simulink model "ARDroneFly_035"  (R2014b)
settings: Solver=FixedStepDiscrete  StartTime=0.0  StopTime=600  FixedStep=1/400  RelTol=1e-3
InitFcn:
  | AR_DRONE_SCRIPT;
  | ControllerDesign;
  | parameters;
values from neighbouring files (symbols this model uses):
  Ah = [0 1; 0 0]    [ControllerDesign.m]
  Axy = [0 1; 0 0]    [ControllerDesign.m]
  C = (eval(C))    [ControllerDesign.m]
  Ch = [1 0]    [ControllerDesign.m]
  Cxy = [1 0]    [ControllerDesign.m]
  Lh = Lh'    [ControllerDesign.m]
  Lxy = Lxy'    [ControllerDesign.m]
  par_g = par.g    [parameters.m]
  par_m = par.m    [parameters.m]
  tauToPwmbar = inv(pwmbarToTau)    [ControllerDesign.m]
undefined symbols (not defined in the file or in its folder): meter, par
libraries: simulink x6, AR_Drone_2_Library x5, dspnetwork x1
(part 1 of 2)
settings Model: SimulationMode=external  ExtModeTrigDuration=120003  Creator=darenlee  LastModifiedBy=s136047
settings OptimizationCC: OptimizeModelRefInitCode=on  LifeSpan=1  MaxStackSize=64
settings DebuggingCC: UnderspecifiedInitializationDetection=Classic  MergeDetectMultiDrivingBlocksExec=none
settings HardwareCC: ProdLargestAtomicInteger=Long  ProdLargestAtomicFloat=Double  ProdEndianess=LittleEndian  ProdHWDeviceType=ARM Compatible->ARM Cortex
settings RTWCC: SystemTargetFile=ert.tlc  TLCOptions=-aInlineSetEventsForThisBaseRateFcn=TLC_FALSE -aSuppressMultiTaskScheduler=TLC_FALSE  TemplateMakefile=ert_default_tmf  Description=Embedded Coder  ProcessScript=ert_make_rtw_hook  Toolchain=Code Sourcery
settings CodeAppCC: IgnoreCustomStorageClasses=off
settings ERTTargetCC: ExtMode=on  ExtModeMexArgs='192.168.1.1' 1 17725

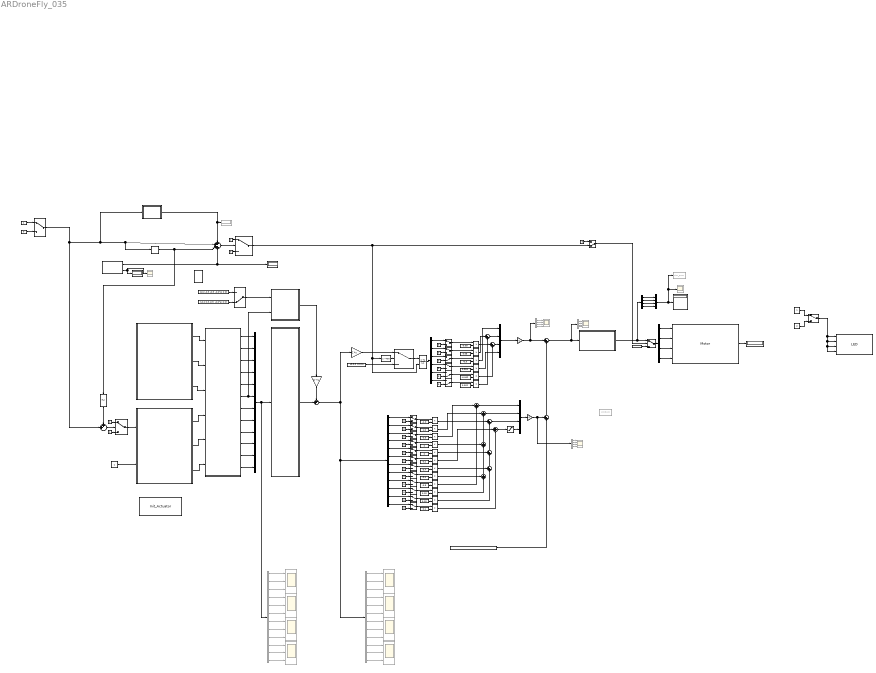
== system ARDroneFly_035 ==
  note: This version is not yet optimal, but some parts work, sorry.
      |
      | Based on: https://github.com/darenlee/SimulinkARDroneTarget
      |
      | Take off
      | 1) Make sure external camera feedback is activated in another Matlab Window (UDP Connection)
      | 2) Activate Green Manual Switch (will only take effect on rising edge)
      | 3) "Take off" signal is 2 seconds delayed, in this time the sensors are calibrated
      | 4) Quad fly's to the the setpoint (blue button)
      |
      | Stop
      | 1) Deactivate Green Manual Switch
      | 2) Quad falls out of the air
      |
      | Low voltage
      | 1) once the voltage has dropped once under the 9 volt the quad will not takeoff again
      | 2) or reset manually in the 'battery check' block
      |
      | Tips to tune the quad
      | 1) deactivate all feedback (manual switches) except for the z, roll, pitch and omega_xyz control
      | 2) test if the quad is some kind of stable (if not then change the gains) (first roll and pitch then omega_xy (omega functions as a differential action (damping)))
      | 3) try to manage that the quad takes off vertically by changing the gravity compensation term
      | 4) tune the rest of the proportional part
      | 5) activate and tune the integral part (be gentle with this one)
      | 6) have a look at the lowpass, luenberger observers (X-Y pos), and the complementary sensor fusion (accel gyro)
  note: [ T_0 TauX_0 TauY_0 TauZ_0 ]
  note: Integral action
  note: Setpoint [ x y z yaw u v ] (in inertia frame)
      | Note: Z must be negative because
      | of NED coordinates
  note: Delay is  added to
      | start integration action only
      | when quad is in the air
  note: Proportional action
  note: Gravity compensation
  0 when battery dropped once under 9 volt 1 when battery OK : Display
  Accel_Norm1 : Scope  Commented=on
      settings: ShowLegends=on  YMin=0  YMax=90  SaveName=Accel_P1
  Accel_Norm10 : Scope  Commented=on  NumInputPorts=4
      settings: ShowLegends=on  YMin=0~-1~-1~-1  YMax=20~1~1~1  SaveName=Accel_P15
  Accel_Norm{2..4,6,8..9,11..12} (8 alike) : Scope  Commented=on  NumInputPorts=3
      Accel_Norm11 settings: YMin=-0.4~-0.4~-0.5  YMax=0.2~0.4~0.2  SaveName=Accel_P2
      Accel_Norm12 settings: YMin=-0.8~-0.6~-0.4  YMax=1.2~0.6~0.4  SaveName=Accel_P7
      Accel_Norm2 settings: YMin=-0.5~-0.4~-0.235  YMax=0.3~0.5~-0.195  SaveName=Accel_P8
      Accel_Norm3 settings: YMin=-0.5~-0.4~0.25  YMax=0.5~0.5~0.5  SaveName=Accel_P
      Accel_Norm4 settings: YMin=-1~-1~-1.5  YMax=1~1~2  SaveName=Accel_P10
      Accel_Norm6 settings: YMin=-1~-1~-1.5  YMax=1~1~2  SaveName=Accel_P3
      Accel_Norm8 settings: YMin=-0.4~-0.4~-0.5  YMax=0.2~0.4~0.2  SaveName=Accel_P4
      Accel_Norm9 settings: YMin=-0.8~-0.6~-0.4  YMax=1.2~0.6~0.4  SaveName=Accel_P6
  Accel_Norm13 : Scope  Commented=on  NumInputPorts=4
      settings: ShowLegends=on  YMin=-0.5~-0.15~-0.15~-0.2  YMax=0.2~0.1~0.15~0.2  SaveName=Accel_P18
  Accel_Norm14 : Scope  Commented=on  NumInputPorts=4
      settings: ShowLegends=on  YMin=3.7~-0.25~-0.5~-0.15  YMax=4.2~0.1~1.5~0.05  SaveName=Accel_P19
  Accel_Norm7 : Scope  Commented=on
      settings: YMin=9  YMax=12  SaveName=Accel_P11
  Battery Check : Subsystem
  Constant{,7..8,10,57} (5 alike) : Constant
  Constant1 : Constant  Value=2
  Constant{5,9,12,30,39..53,56,59,61} (22 alike) : Constant  Value=0
  Constant13 : Constant  Value=[0 0 0 0]
  Constant14 : Constant  Value=-1.0
  Constant15 : Constant  Value=1.0
  Constant16 : Constant  Value=-0.9
  Constant17 : Constant  Value="[-0.2 -0.3 -0.5  -0.0*pi 0 0]"
  Constant2 : Constant  Value=0.4
  Constant20 : Constant  Value=2
  Constant21 : Constant  Value=2
  Constant22 : Constant  Value=0.2
  Constant23 : Constant  Value=-0.4
  Constant24 : Constant  Value="[1.1*par_m*par_g      -0.02     -0.083    -0.027]"
  Constant27 : Constant  Value=-0.05
  Constant28 : Constant  Value=0.05
  Constant29 : Constant  Value=-0.5
  Constant3 : Constant  Value="[-0.2 0.3 -0.5  -0.0*pi 0 0]"
  Constant32 : Constant  Value=0.004
  Constant33 : Constant  Value=0.15
  Constant34 : Constant  Value=0.15
  Constant35 : Constant  Value=0.1
  Constant58 : Constant  Value=-0.002
  Constant6 : Constant  Value=-0.5
  Constant60 : Constant  Value=0.002
  Constant62 : Constant  Value="[0 0 0  0 0 0]"
  Delay1 : Delay  DelayLength=800  InitialCondition=0
  Delay3 : Delay  DelayLength=400  InitialCondition=0
  Demux1 : Demux  Commented=on  Outputs=12
  Demux10 : Demux  Commented=on
  Demux11 : Demux  Commented=on
  Demux12 : Demux  Commented=on
  Demux3 : Demux  Commented=on  Outputs=12
  Demux4 : Demux
  Demux5 : Demux
  Demux8 : Demux  Outputs=12
  Demux9 : Demux  Outputs=6
  Discrete-Time Integrator1 : DiscreteIntegrator  ExternalReset=rising  InitialConditionSetting=State (most efficient)  SampleTime=-1
  Gain2 : Gain  Gain=C'  Multiplication=Matrix(K*u)
  Gain6 : Gain  Gain=C  Multiplication=Matrix(K*u)  SampleTime=0.0025
  Init_Actuator : AR_Drone_2_Library/Init_Actuator  ShowSpec=on
  Invert Signal : Fcn  Expr=-(u(1)-1)
  LED : AR_Drone_2_Library/LED
  Low Pass Filters and Luenberg Observers : Subsystem
  Mag1 : Display
  Manual Switch{3..16,18} (15 alike) : ManualSwitch
  Manual Switch{17,19..21} (4 alike) : ManualSwitch  CurrentSetting=0
  Motor : AR_Drone_2_Library/Motor
  Motor Thrust/Torque model : Subsystem
  Mux14 : Mux
  Mux15 : Mux
  Mux4 : Mux  Inputs=12
  Mux6 : Mux
  Negative gain feedback : Gain  Gain=-1
  Negative integral feedback : Gain  Gain=-1
  Product{1..3,7..10,12..22} (18 alike) : Product
  "Sensor Measurements, Low Pass Filter, Calibrations, and Corrections " : Subsystem
  Set and hold after first rising edge : Subsystem
  Setpoint To Pilot Frame : Subsystem
  "Shut off pwm output (debug purpose) " : ManualSwitch  CurrentSetting=0
  States To Pilot Frame : Subsystem
  Sum{1..2,5,10,12,16,22} (7 alike) : Sum  Inputs=|++
  Sum{8,17..21} (6 alike) : Sum  Inputs=++|
  Sum3 : Sum  Inputs=++++
  Sum7 : Sum  Inputs=-+|
  Switch : Switch  Criteria=u2 > Threshold
  Switch1 : Switch  Threshold=4
  Switch3 : Switch  Threshold=2
  Switch4 : Switch  Threshold=1
  Switch6 : Switch  Criteria=u2 > Threshold
  Take off and shutdown (reacts only at rising edges) : ManualSwitch
  To Workspace4 : ToWorkspace  Commented=on  VariableName=simPwm  SampleTime=-1
  To Workspace7 : ToWorkspace  Commented=on  VariableName=sim_pwm  SaveFormat=Timeseries  SampleTime=-1
  Volt : Display
  Volt3 : Display  Commented=on
  We lost too much thrust if we dont do this (gain too high) : Saturate  UpperLimit=0.1  LowerLimit=-0.1
  from topcam via UDP : Subsystem
  track yaw : Subsystem
  ydf1 : Display
  wires:
  Switch/1 -> LED/4, LED/3, LED/2, LED/1
  Motor/1 -> Mag1/1
  Switch3/1 -> "Sensor Measurements, Low Pass Filter, Calibrations, and Corrections "/1(Hold Calibration Signal)
  Constant7/1 -> "Sensor Measurements, Low Pass Filter, Calibrations, and Corrections "/2(Activate Calibration Accel Angles)
  Switch1/1 -> Discrete-Time Integrator1/2, Delay3/1, "Shut off pwm output (debug purpose) "/2
  Constant5/1 -> Switch1/3
  Constant8/1 -> Switch1/1
  Constant9/1 -> Take off and shutdown (reacts only at rising edges)/2
  Constant10/1 -> Take off and shutdown (reacts only at rising edges)/1
  Sum3/1 -> Switch1/2
  Battery Check/1(Battery Volt OK) -> 0 when battery dropped once under 9 volt 1 when battery OK/1, Sum3/4
  Battery Check/2(volt) -> Volt/1, Accel_Norm7/1
  Demux4/2 -> Mux6/2  "2"
  Demux4/1 -> Mux6/1  "1"
  Demux4/3 -> Mux6/3  "3"
  Demux4/4 -> Mux6/4  "4"
  Mux6/1 -> To Workspace7/1, Accel_Norm1/1, ydf1/1
  "Shut off pwm output (debug purpose) "/1 -> Switch6/2
  Constant12/1 -> "Shut off pwm output (debug purpose) "/1
  Switch6/1 -> Demux5/1
  Constant13/1 -> Switch6/3
  Demux5/4 -> Motor/4  "4"
  Demux5/3 -> Motor/3  "3"
  Demux5/2 -> Motor/2  "2"
  Demux5/1 -> Motor/1  "1"
  "Sensor Measurements, Low Pass Filter, Calibrations, and Corrections "/2(Roll Pitch (Integrated Gyro + Accel Corrected)) -> Low Pass Filters and Luenberg Observers/5(roll pitch_in)
  "Sensor Measurements, Low Pass Filter, Calibrations, and Corrections "/3(Gyro omega_xyz) -> Low Pass Filters and Luenberg Observers/6(wx wy wz_ in)
  "Sensor Measurements, Low Pass Filter, Calibrations, and Corrections "/1(Height UltraSound) -> Low Pass Filters and Luenberg Observers/4(z_in)
  Constant14/1 -> Product1/2
  Constant15/1 -> Product2/2
  Constant16/1 -> Product3/2
  Constant20/1 -> Product7/2
  Constant21/1 -> Product8/2
  Constant22/1 -> Product9/2
  Constant23/1 -> Product10/2
  Sum1/1 -> Mux14/1  "T"
  Sum5/1 -> Mux14/3  "tau_y"
  Sum2/1 -> Mux14/2  "tau_x"
  Mux14/1 -> Negative gain feedback/1
  Constant24/1 -> Sum20/2
  Constant27/1 -> Product12/2
  Constant28/1 -> Product13/2
  Constant29/1 -> Product14/2
  Discrete-Time Integrator1/1 -> Demux9/1
  Sum20/1 -> Sum12/2
  Sum12/1 -> Motor Thrust/Torque model/1("[ T tau_xyz ]"), Demux12/1
  Mux15/1 -> Negative integral feedback/1
  Constant32/1 -> Product15/2
  Negative integral feedback/1 -> Sum12/1, Demux10/1
  Demux10/1 -> Accel_Norm10/1
  Demux10/4 -> Accel_Norm10/4
  Demux10/3 -> Accel_Norm10/3
  Demux10/2 -> Accel_Norm10/2
  Negative gain feedback/1 -> Demux11/1, Sum20/1
  Demux11/1 -> Accel_Norm13/1
  Demux11/4 -> Accel_Norm13/4
  Demux11/3 -> Accel_Norm13/3
  Demux11/2 -> Accel_Norm13/2
  Demux12/1 -> Accel_Norm14/1
  Demux12/4 -> Accel_Norm14/4
  Demux12/3 -> Accel_Norm14/3
  Demux12/2 -> Accel_Norm14/2
  from topcam via UDP/1(real x) -> Low Pass Filters and Luenberg Observers/1(x_in)
  from topcam via UDP/2("real y ") -> Low Pass Filters and Luenberg Observers/2(y_in)
  from topcam via UDP/3(real psi) -> Low Pass Filters and Luenberg Observers/3(yaw_in)
  Constant2/1 -> Product17/2
  Constant6/1 -> Product18/2
  Constant33/1 -> Product19/2
  Constant34/1 -> Product20/2
  Constant35/1 -> Product16/2
  Demux8/2 -> Manual Switch4/1  "y"
  Demux8/3 -> Manual Switch5/1  "z"
  Demux8/1 -> Manual Switch3/1  "x"
  Demux8/6 -> Manual Switch8/1  "yaw"
  Sum16/1 -> We lost too much thrust if we dont do this (gain too high)/1
  Product18/1 -> Sum1/2
  Product19/1 -> Sum17/2
  Product17/1 -> Sum17/1
  Product20/1 -> Sum18/2
  Product10/1 -> Sum18/1  "tau_z"
  Product9/1 -> Sum16/1
  Product1/1 -> Sum5/1
  Product2/1 -> Sum2/1
  Product3/1 -> Sum1/1
  Sum19/1 -> Sum2/2
  Sum17/1 -> Sum19/2
  Product7/1 -> Sum19/1
  Sum21/1 -> Sum5/2
  Sum18/1 -> Sum21/2
  Product8/1 -> Sum21/1
  Manual Switch3/1 -> Product1/1
  Constant39/1 -> Manual Switch3/2
  Constant40/1 -> Manual Switch4/2
  Constant41/1 -> Manual Switch5/2
  Constant42/1 -> Manual Switch6/2
  Constant43/1 -> Manual Switch7/2
  Constant44/1 -> Manual Switch8/2
  Constant45/1 -> Manual Switch9/2
  Constant46/1 -> Manual Switch10/2
  Constant47/1 -> Manual Switch11/2
  Constant48/1 -> Manual Switch12/2
  Constant49/1 -> Manual Switch13/2
  Constant50/1 -> Manual Switch14/2
  Demux8/12 -> Manual Switch14/1  "omega z"
  Demux8/11 -> Manual Switch13/1  "omega y"
  Demux8/10 -> Manual Switch12/1  "omega x"
  Demux8/9 -> Manual Switch11/1  "w"
  Demux8/8 -> Manual Switch10/1  "v"
  Demux8/7 -> Manual Switch9/1  "u"
  Demux8/5 -> Manual Switch7/1  "pitch"
  Demux8/4 -> Manual Switch6/1  "roll"
  Manual Switch14/1 -> Product16/1
  Manual Switch13/1 -> Product20/1
  Manual Switch12/1 -> Product19/1
  Manual Switch11/1 -> Product18/1
  Manual Switch10/1 -> Product17/1
  Manual Switch9/1 -> Product10/1
  Manual Switch8/1 -> Product9/1
  Manual Switch7/1 -> Product8/1
  Manual Switch6/1 -> Product7/1
  Manual Switch5/1 -> Product3/1
  Manual Switch4/1 -> Product2/1
  Product14/1 -> Mux15/1  "T"
  Product15/1 -> Mux15/4  "tau_z"
  Constant30/1 -> Manual Switch15/2
  Constant51/1 -> Manual Switch16/2
  Constant52/1 -> Manual Switch17/2
  Constant53/1 -> Manual Switch18/2
  Manual Switch18/1 -> Product15/1
  Demux9/4 -> Manual Switch18/1  "yaw"
  Manual Switch17/1 -> Product14/1
  Demux9/3 -> Manual Switch17/1  "z"
  Demux9/2 -> Manual Switch16/1  "y"
  Manual Switch16/1 -> Product13/1
  Manual Switch15/1 -> Product12/1
  Demux9/1 -> Manual Switch15/1  "x"
  Constant1/1 -> Switch/3
  Constant/1 -> Switch/1
  Delay1/1 -> Sum3/3, Invert Signal/1
  Constant56/1 -> Switch3/1
  Constant57/1 -> Switch3/3
  Set and hold after first rising edge/1(Out) -> Volt3/1, Sum3/1
  Take off and shutdown (reacts only at rising edges)/1 -> Sum8/2, Delay1/1, Sum3/2, Set and hold after first rising edge/1(In)
  Constant58/1 -> Product21/2
  Constant59/1 -> Manual Switch19/2
  Manual Switch19/1 -> Product21/1
  Demux9/5 -> Manual Switch19/1  "u"
  Constant60/1 -> Product22/2
  Constant61/1 -> Manual Switch20/2
  Manual Switch20/1 -> Product22/1
  Demux9/6 -> Manual Switch20/1  "v"
  Sum10/1 -> Mux15/3  "tau_y"
  Product12/1 -> Sum10/1  "tau_y"
  Product21/1 -> Sum10/2
  Sum22/1 -> Mux15/2  "tau_x"
  Product13/1 -> Sum22/1  "tau_x"
  Product22/1 -> Sum22/2
  Switch4/1 -> Discrete-Time Integrator1/1
  Sum8/1 -> Switch3/2
  Invert Signal/1 -> Sum8/1
  Delay3/1 -> Switch4/2
  Demux1/1 -> Accel_Norm3/1
  Demux1/2 -> Accel_Norm3/2
  Demux1/3 -> Accel_Norm3/3
  Demux1/4 -> Accel_Norm6/1
  Demux1/5 -> Accel_Norm6/2
  Demux1/6 -> Accel_Norm6/3
  Demux1/7 -> Accel_Norm8/1
  Demux1/8 -> Accel_Norm8/2
  Demux1/9 -> Accel_Norm8/3
  Demux1/10 -> Accel_Norm9/1
  Demux1/11 -> Accel_Norm9/2
  Demux1/12 -> Accel_Norm9/3
  Low Pass Filters and Luenberg Observers/1(x_out) -> Mux4/1
  Low Pass Filters and Luenberg Observers/2(y_out) -> Mux4/2
  Low Pass Filters and Luenberg Observers/3(z_out) -> Mux4/3
  Low Pass Filters and Luenberg Observers/4(roll_out) -> Mux4/4
  Low Pass Filters and Luenberg Observers/5(pitch_out) -> Mux4/5
  Low Pass Filters and Luenberg Observers/6(yaw out) -> Setpoint To Pilot Frame/2(yaw), Mux4/6
  Low Pass Filters and Luenberg Observers/7(u_out) -> Mux4/7
  Low Pass Filters and Luenberg Observers/8(v_out) -> Mux4/8
  Low Pass Filters and Luenberg Observers/9(w_out) -> Mux4/9
  Low Pass Filters and Luenberg Observers/10(omega x_out) -> Mux4/10
  Low Pass Filters and Luenberg Observers/11(omega y_out) -> Mux4/11
  Low Pass Filters and Luenberg Observers/12(omega z_out) -> Mux4/12
  Mux4/1 -> Demux3/1, States To Pilot Frame/1(State)
  Gain6/1 -> Switch4/1
  Constant62/1 -> Switch4/3
  Demux3/1 -> Accel_Norm2/1
  Demux3/2 -> Accel_Norm2/2
  Demux3/3 -> Accel_Norm2/3
  Demux3/4 -> Accel_Norm4/1
  Demux3/5 -> Accel_Norm4/2
  Demux3/6 -> Accel_Norm4/3
  Demux3/7 -> Accel_Norm11/1
  Demux3/8 -> Accel_Norm11/2
  Demux3/9 -> Accel_Norm11/3
  Demux3/10 -> Accel_Norm12/1
  Demux3/11 -> Accel_Norm12/2
  Demux3/12 -> Accel_Norm12/3
  States To Pilot Frame/1(State pilot frame) -> Sum7/2
  Gain2/1 -> Sum7/1
  Setpoint To Pilot Frame/1(Setpoint pilot frame) -> Gain2/1
  Sum7/1 -> Demux1/1, Demux8/1, Gain6/1  "Error Signal"
  Product16/1 -> Sum16/2
  We lost too much thrust if we dont do this (gain too high)/1 -> Mux14/4
  Motor Thrust/Torque model/1(PWM_1,2,3,4) -> Switch6/1, Demux4/1
  Constant17/1 -> Manual Switch21/1
  Constant3/1 -> Manual Switch21/2
  Manual Switch21/1 -> Setpoint To Pilot Frame/1(Setpoint)

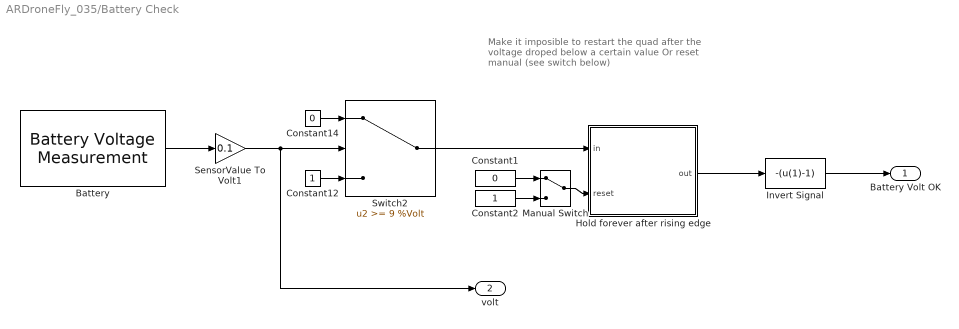
== system ARDroneFly_035/Battery Check ==
  note: Make it imposible to restart the quad
      | after the voltage droped below a certain value
      |
      | Or reset manual (see switch below)
  Battery : AR_Drone_2_Library/Battery Voltage Measurement  SFunctionSpec=void BatteryMeasure_step(single y1[1])  SampleTime=-1
  Constant1 : Constant  Value=0
  Constant12 : Constant
  Constant14 : Constant  Value=0
  Constant2 : Constant
  Hold forever after rising edge : Subsystem
  Invert Signal : Fcn  Expr=-(u(1)-1)
  Manual Switch : ManualSwitch
  SensorValue To Volt1 : Gain  Gain=0.1
  Switch2 : Switch  Threshold=9 %Volt
  Battery Volt OK : Outport
  volt : Outport  Port=2
  wires:
  Constant14/1 -> Switch2/1
  Constant12/1 -> Switch2/3
  Battery/1 -> SensorValue To Volt1/1
  SensorValue To Volt1/1 -> volt/1, Switch2/2
  Switch2/1 -> Hold forever after rising edge/1(in)
  Hold forever after rising edge/1(out) -> Invert Signal/1
  Constant1/1 -> Manual Switch/1
  Constant2/1 -> Manual Switch/2
  Manual Switch/1 -> Hold forever after rising edge/2(reset)
  Invert Signal/1 -> Battery Volt OK/1

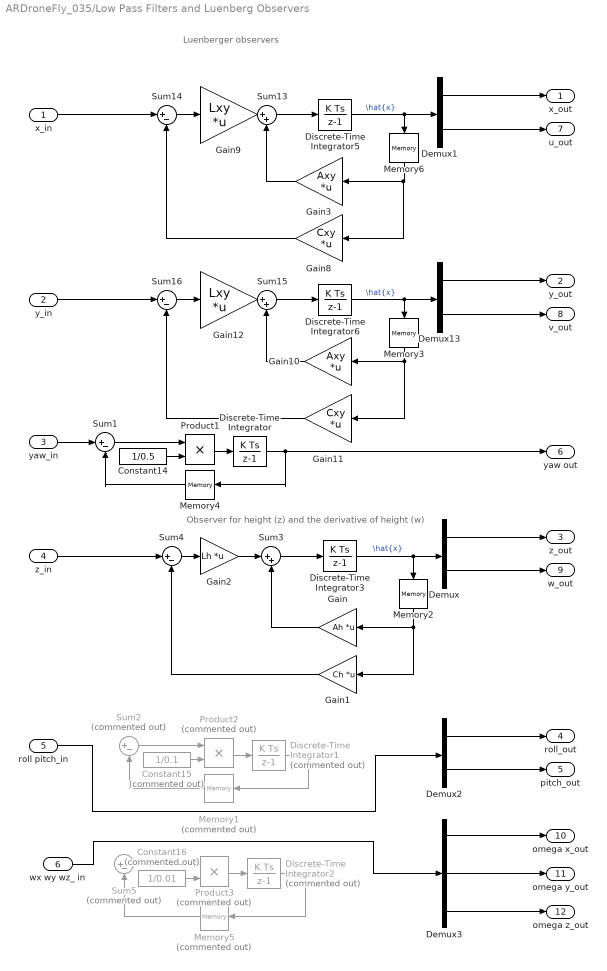
== system ARDroneFly_035/Low Pass Filters and Luenberg Observers ==
  note: Luenberger observers
  note: Observer for height (z) and the derivative of height (w)
  x_in : Inport
  y_in : Inport  Port=2
  yaw_in : Inport  Port=3
  z_in : Inport  Port=4
  roll pitch_in : Inport  Port=5
  wx wy wz_ in : Inport  Port=6
  Constant14 : Constant  Value=1/0.5
  Constant15 : Constant  Commented=on  Value=1/0.1
  Constant16 : Constant  Commented=on  Value=1/0.01
  Demux{,1..2,13} (4 alike) : Demux  Outputs=2
  Demux3 : Demux  Outputs=3
  Discrete-Time Integrator : DiscreteIntegrator  InitialConditionSetting=State (most efficient)  SampleTime=-1
  Discrete-Time Integrator1 : DiscreteIntegrator  Commented=on  InitialConditionSetting=State (most efficient)  SampleTime=-1
  Discrete-Time Integrator2 : DiscreteIntegrator  Commented=on  InitialConditionSetting=State (most efficient)  SampleTime=-1
  Discrete-Time Integrator3 : DiscreteIntegrator  InitialCondition=[0 0]  InitialConditionSetting=State (most efficient)  SampleTime=-1
  Discrete-Time Integrator5 : DiscreteIntegrator  InitialCondition=[0 0]  InitialConditionSetting=State (most efficient)  SampleTime=-1
  Discrete-Time Integrator6 : DiscreteIntegrator  InitialCondition=[0 0]  InitialConditionSetting=State (most efficient)  SampleTime=-1
  Gain : Gain  Gain=Ah  Multiplication=Matrix(K*u)
  Gain1 : Gain  Gain=Ch  Multiplication=Matrix(K*u)
  Gain10 : Gain  Gain=Axy  Multiplication=Matrix(K*u)
  Gain11 : Gain  Gain=Cxy  Multiplication=Matrix(K*u)
  Gain12 : Gain  Gain=Lxy  Multiplication=Matrix(K*u)
  Gain2 : Gain  Gain=Lh  Multiplication=Matrix(K*u)
  Gain3 : Gain  Gain=Axy  Multiplication=Matrix(K*u)
  Gain8 : Gain  Gain=Cxy  Multiplication=Matrix(K*u)
  Gain9 : Gain  Gain=Lxy  Multiplication=Matrix(K*u)
  Memory1 : Memory  Commented=on
  Memory{2..4,6} (4 alike) : Memory
  Memory5 : Memory  Commented=on
  Product1 : Product
  Product2 : Product  Commented=on
  Product3 : Product  Commented=on
  Sum{1,4,14,16} (4 alike) : Sum  Inputs=|+-
  Sum13 : Sum  Inputs=|++
  Sum15 : Sum  Inputs=|++
  Sum2 : Sum  Commented=on  Inputs=|+-
  Sum3 : Sum  Inputs=|++
  Sum5 : Sum  Commented=on  Inputs=|+-
  x_out : Outport
  y_out : Outport  Port=2
  z_out : Outport  Port=3
  roll_out : Outport  Port=4
  pitch_out : Outport  Port=5
  yaw out : Outport  Port=6
  u_out : Outport  Port=7
  v_out : Outport  Port=8
  w_out : Outport  Port=9
  omega x_out : Outport  Port=10
  omega y_out : Outport  Port=11
  omega z_out : Outport  Port=12
  wires:
  yaw_in/1 -> Sum1/1
  Sum1/1 -> Product1/1
  Discrete-Time Integrator/1 -> yaw out/1, Memory4/1
  Discrete-Time Integrator2/1 -> Memory5/1
  Discrete-Time Integrator1/1 -> Memory1/1
  Product1/1 -> Discrete-Time Integrator/1
  Constant14/1 -> Product1/2
  Product2/1 -> Discrete-Time Integrator1/1
  Sum2/1 -> Product2/1
  Constant15/1 -> Product2/2
  Product3/1 -> Discrete-Time Integrator2/1
  Constant16/1 -> Product3/2
  Sum5/1 -> Product3/1
  z_in/1 -> Sum4/1
  Discrete-Time Integrator3/1 -> Demux/1, Memory2/1  "\\hat{x}"
  Sum3/1 -> Discrete-Time Integrator3/1
  Demux/1 -> z_out/1
  Demux/2 -> w_out/1
  Sum4/1 -> Gain2/1
  Gain1/1 -> Sum4/2
  Gain/1 -> Sum3/2
  Gain2/1 -> Sum3/1
  x_in/1 -> Sum14/1
  Discrete-Time Integrator5/1 -> Demux1/1, Memory6/1  "\\hat{x}"
  Sum13/1 -> Discrete-Time Integrator5/1
  Demux1/1 -> x_out/1
  Demux1/2 -> u_out/1
  Sum14/1 -> Gain9/1
  Gain8/1 -> Sum14/2
  Gain3/1 -> Sum13/2
  Gain9/1 -> Sum13/1
  y_in/1 -> Sum16/1
  Discrete-Time Integrator6/1 -> Demux13/1, Memory3/1  "\\hat{x}"
  Sum15/1 -> Discrete-Time Integrator6/1
  Demux13/1 -> y_out/1
  Demux13/2 -> v_out/1
  Sum16/1 -> Gain12/1
  Gain11/1 -> Sum16/2
  Gain10/1 -> Sum15/2
  Gain12/1 -> Sum15/1
  Demux2/1 -> roll_out/1
  Demux2/2 -> pitch_out/1
  Demux3/1 -> omega x_out/1
  Demux3/2 -> omega y_out/1
  Demux3/3 -> omega z_out/1
  Memory5/1 -> Sum5/2
  Memory1/1 -> Sum2/2
  Memory2/1 -> Gain/1, Gain1/1
  Memory3/1 -> Gain10/1, Gain11/1
  Memory4/1 -> Sum1/2
  Memory6/1 -> Gain8/1, Gain3/1
  roll pitch_in/1 -> Demux2/1
  wx wy wz_ in/1 -> Demux3/1

== system ARDroneFly_035/Motor Thrust//Torque model ==
  note: Motor thrust/torque model:
      |
      |   T_i   = c_m*(pwm_i + k)^2
      |  tau_i = d_m*(pwm_i + k)^2
      |
      | where i is the motor number
  note: There are story's on the internet that a too high current
      |  can damage the motors, therefore we limit the signal
      |
      | Also avoid zero because the behavior between 0 (motor off)
      | and 1 (=approx 5%) is not smooth
  "[ T tau_xyz ]" : Inport
  Constant4 : Constant  Value=par.k
  Inverse of the decouple matrix : Gain  Gain=tauToPwmbar  Multiplication=Matrix(K*u)
  Saturation4 : Saturate  UpperLimit=85  LowerLimit=2
  Sqrt : Sqrt  SaturateOnIntegerOverflow=on
  Sum4 : Sum  Inputs=|+-
  avoid negative values : Saturate  UpperLimit=inf  LowerLimit=0
  PWM_1,2,3,4 : Outport
  wires:
  Sqrt/1 -> Sum4/1
  Constant4/1 -> Sum4/2
  Sum4/1 -> Saturation4/1
  avoid negative values/1 -> Sqrt/1
  Saturation4/1 -> PWM_1,2,3,4/1
  Inverse of the decouple matrix/1 -> avoid negative values/1
  "[ T tau_xyz ]"/1 -> Inverse of the decouple matrix/1

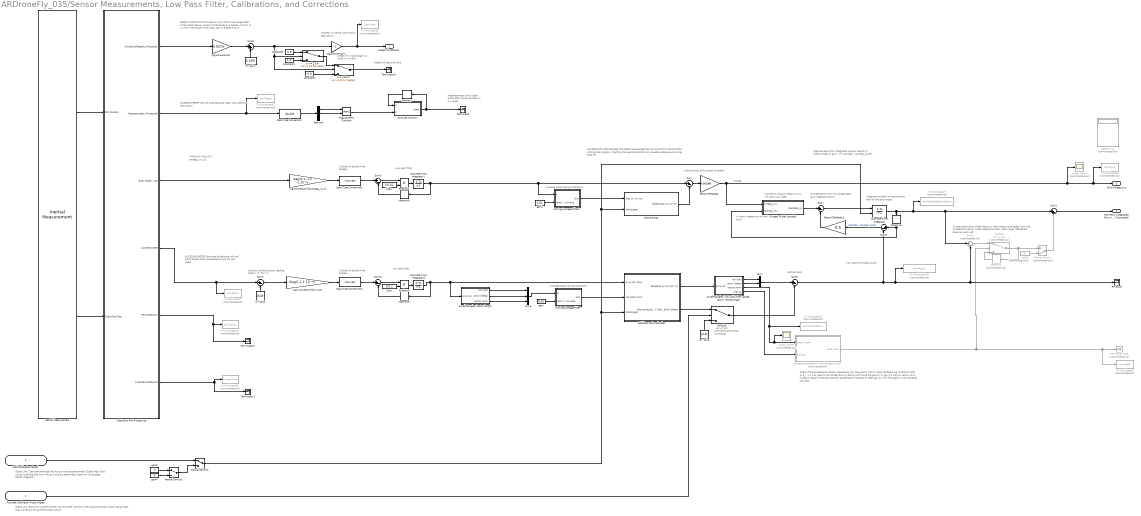
== system ARDroneFly_035/Sensor Measurements, Low Pass Filter, Calibrations, and Corrections  ==
  note: omega
  note: [roll, pitch] (lambda Accel)
  note: Remove Bias from integrated angular velocity's
      | d/dt*Lambda = gyro - k*(Llambda - Lambda_accel)
  note: Compensation term to
      | compensate  gyro integration error
  note: Q matrix depent
      | on roll and pitch
  note: Active/not active
      | bias correction
  note: Signal Low: Bias from accelerometer not removed (use this when quad on gimbal stand)
      | Signal High: Bias correction on accelerometer active
  note: Signal Low: Calculate average bias  for gyro and accelerometer
      | Signal High: Bias values undo the bias from the gyro and accelerometer
      | Signal on rising edge: Reset integrator
  note: Average signal during calibration
  note: Low pass filter
  note: Convert to double
      | if not already
  note: Magnetometer yaw
      | (signal drops after some
      | seconds on my quad)
  note: Height Ultrasound Valid
  note: Express in inertia frame
      | North East Down
  note: Transform Angular velocitiy's
      | to roll pitch yaw rates
  note: Check if the acceleration sensor represents only the gravity
      | This is when the following conditions hold
      | 1)   a_z >= 0	   % quad is not upside down or falling with twice the gravity
      | 2)  ||a|| == 9.81     % vector norm is approx equal to the gravitational acceleration constant
      | 3)  d/dt*||a|| == 0   % the signal is not changing very fast
  note: subtract bias
  note: subtract bias and convert to radials
  note: subtract half the sensor reading
      | 2048 = (2^12) / 2
  note: ACCELEROMETER
      | Estimate of absolute roll and pitch angles
      | (body accelerations are not yet used)
  note: Correct estimation when there is a valid measure
      | of angles from the Acceleratio sensor (undo integration bias)
      | (Hard reset, Tested but does not work yet)
  note: Integrate to obtain an estimate
      | for the roll and pitch angle
  note: CALIBRATION PROCEDURE
      | calculates  the average bias  during the first second after starting the program,
      | therfore the quad should start at a leveled underground during take off
  note: ANGULAR VELOCITY
      | omega_{x,y,z}
  note: MAGNETOMETER
      | not yet used because highly disturbed by the motors
  note: HEIGHT APPROXIMATION
      | Sensor only valid in the range 0.997 - 2.750 meter
      | Sensor value 0 corresponds to a height <0.20 m or >2.75 m
      | The slope in the linear part is 0.0076 m/unit
  note: Check if in Valid range
      | 1 = valid
      | 0 = invalid
  note: Convert to double
      | if not already
  note: Low pass filter
  note: Average signal during calibration
  Hold Calibration Signal : Inport
  Activate Calibration Accel Angles : Inport  Port=2
  (2^12)/1 : Constant  Value=0.1997
  (2^12)/2 : Constant  Value=2048
  (2^12)/3 : Constant  Value=[0;0]
  1/tau : Constant  Value=1/0.2
  "1/tau " : Constant  Value=1/0.01
  AccelToAngles Vector length : Subsystem
  AccelToAngles (not valid when upside down) VectorLength : Subsystem
  Accel_Norm4 : Scope  Commented=on
      settings: YMin=-3  YMax=4  SaveName=Accel_P5
  Accel_Norm6 : Scope  Commented=on
      settings: YMin=0  YMax=16  SaveName=Accel_P12
  CheckSum Pre-Processing : Subsystem
  Constant1 : Constant  Value=1.0
  Constant2 : Constant  Value=0.0
  Constant5 : Constant  Value=0.0
  Data Type Conversion : DataTypeConversion  OutDataTypeStr=double
  Data Type Conversion1 : DataTypeConversion
  Data Type Conversion2 : DataTypeConversion
  Demux4 : Demux  Outputs=3
  Discrete-Time Integrator : DiscreteIntegrator  ExternalReset=rising  InitialCondition=[0 0 ]  InitialConditionSetting=State (most efficient)  SampleTime=-1
  Discrete-Time Integrator1 : DiscreteIntegrator  InitialConditionSetting=State (most efficient)  SampleTime=-1
  Discrete-Time Integrator3 : DiscreteIntegrator  InitialCondition=[0.1 0.2 0.3]  InitialConditionSetting=State (most efficient)  SampleTime=-1
  Hold bias and scale after : Subsystem
  Hold the bias : Subsystem
  Inertial Measurement : AR_Drone_2_Library/Inertial Measurement  Ts=1/400
  MATLAB Function : MATLAB Function  TreatAsAtomicUnit=on
  Manual Switch : ManualSwitch  Commented=on  CurrentSetting=0
  Manual Switch1 : ManualSwitch
  Manual Switch2 : ManualSwitch
  Memory : Memory
  Memory2 : Memory  Commented=on  X0=[0 0]
  Memory3 : Memory  X0=[0.01 0.01 0.01]
  Memory4 : Memory  X0=[0.01 0.01 0.01]
  Memory6 : Memory  X0=[0.0 0.0]
  Moving Average Filter : Subsystem
  Moving Average Filter1 : Subsystem
  Mux1 : Mux  Inputs=3
  Mux7 : Mux  Inputs=2
  Omega To d/dt Lambda : MATLAB Function  TreatAsAtomicUnit=on
  OptFlow V3 : Display  Commented=on
  Product2 : Product
  Product5 : Product
  RP Accel : Terminator
  RPY Accel Valid : Terminator  Commented=on
  SensorToRadials : Gain  Gain=0.001069
  SensorToRadials1 : Gain  Gain=0.5
  Sum{,1,3..5,7..8,10} (8 alike) : Sum  Inputs=|+-
  Sum2 : Sum  Commented=on  Inputs=|+-
  Sum6 : Sum  Inputs=|++
  Switch2 : Switch  Commented=on  Threshold=0.1
  Switch3 : Switch  Threshold=0.1
  Terminator{,1..3} (4 alike) : Terminator
  To Workspace : ToWorkspace  Commented=on  VariableName=simAccel  SampleTime=-1
  To Workspace1 : ToWorkspace  Commented=on  VariableName=simGyro  SampleTime=-1
  To Workspace10 : ToWorkspace  Commented=on  VariableName=simAccel  SampleTime=-1
  To Workspace2 : ToWorkspace  Commented=on  VariableName=simMagn  SampleTime=-1
  To Workspace3 : ToWorkspace  Commented=on  VariableName=simUltra  SampleTime=-1
  To Workspace4 : ToWorkspace  Commented=on  VariableName=simTemp  SampleTime=-1
  To Workspace5 : ToWorkspace  Commented=on  VariableName=simAccelTemp  SampleTime=-1
  To Workspace7 : ToWorkspace  Commented=on  VariableName=simAttitudeEstimation  SampleTime=-1
  To Workspace8 : ToWorkspace  Commented=on  VariableName=simValid  SampleTime=-1
  To Workspace9 : ToWorkspace  Commented=on  VariableName=simVectorNorm  SampleTime=-1
  Trigonometric Function : Trigonometry  Operator=atan2
  Validate acceleration must be approx 9.81 : Subsystem  Commented=on
  gain : Constant  Value=0.01
  gain1 : Constant  Value=0.01
  gain2 : Constant  Commented=on  Value=0
  gain3 : Constant
  gain4 : Constant  Value=0
  h < 0.20 m : Switch  Criteria=u2 > Threshold  Threshold=0.20 % [meter]
  h >= 2.5 m : Switch  Threshold=2.5 %[meter]
  sign convention flip x axis : Gain  Gain=diag([-1 1 1])  Multiplication=Matrix(K*u)
  "signconvention flip omega_{y,z}" : Gain  Gain=diag([1.0 -1.0 -1.0])  Multiplication=Matrix(K*u)
  signconvention1 : Gain  Gain=-1
  signconvention2 : Gain  Gain=0.0076
  Height UltraSound : Outport
  Roll Pitch (Integrated Gyro + Accel Corrected) : Outport  Port=2
  Gyro omega_xyz : Outport  Port=3
  wires:
  CheckSum Pre-Processing/5(TempMeasure) -> Terminator2/1, To Workspace4/1
  CheckSum Pre-Processing/6(AccelTempMeasure) -> Terminator1/1, To Workspace5/1
  Inertial Measurement/2 -> CheckSum Pre-Processing/2(CheckSumFlag)
  Inertial Measurement/1 -> CheckSum Pre-Processing/1(IMU Packets)
  CheckSum Pre-Processing/4(Accelerometer) -> To Workspace/1, Sum4/1
  CheckSum Pre-Processing/1(UltraSoundHeight_Processed) -> signconvention2/1
  (2^12)/2/1 -> Sum4/2
  gain/1 -> Moving Average Filter/2(ratio new/old value)
  AccelToAngles Vector length/1(roll (phi)) -> Mux1/1
  AccelToAngles Vector length/2(pitch (theta)) -> Mux1/2
  AccelToAngles Vector length/3(vector norm) -> Mux1/3
  Hold bias and scale after/1("Scaled ax ay az [N/s^2] ") -> AccelToAngles (not valid when upside down) VectorLength/1(ax ay az)
  Hold bias and scale after/2("bias correction roll (phi), pitch (theta)") -> Switch3/1
  AccelToAngles (not valid when upside down) VectorLength/3(vector norm) -> To Workspace9/1, Validate acceleration must be approx 9.81/1(vector norm), Accel_Norm6/1
  AccelToAngles (not valid when upside down) VectorLength/4(sign az) -> Validate acceleration must be approx 9.81/2(sign(az))
  Validate acceleration must be approx 9.81/1(accel valid) -> RPY Accel Valid/1, To Workspace8/1, Switch2/2
  CheckSum Pre-Processing/3(Body Rates - pqr) -> "signconvention flip omega_{y,z}"/1
  gain1/1 -> Moving Average Filter1/2(ratio new/old value)
  Moving Average Filter1/1(Out) -> Hold the bias/1(bias wx wy wz)
  Hold the bias/1(" holded bias wx wy wz") -> Sum/2
  Sum/1 -> SensorToRadials/1
  SensorToRadials/1 -> Omega To d/dt Lambda/1(omega_xyz), Accel_Norm4/1, To Workspace1/1, Gyro omega_xyz/1
  Switch2/1 -> Manual Switch/1, Memory2/1
  Memory2/1 -> Switch2/3
  Sum2/1 -> Switch2/1
  signconvention2/1 -> Sum6/1
  (2^12)/1/1 -> Sum6/2
  Sum6/1 -> h < 0.20 m/2, h >= 2.5 m/2, signconvention1/1
  Constant1/1 -> h >= 2.5 m/3
  Constant5/1 -> h >= 2.5 m/1
  Constant2/1 -> h < 0.20 m/3
  h >= 2.5 m/1 -> h < 0.20 m/1
  h < 0.20 m/1 -> Terminator3/1
  CheckSum Pre-Processing/2(Magnetometer_Processed) -> To Workspace2/1, Data Type Conversion/1
  Omega To d/dt Lambda/1(dlambda_rp) -> Sum7/1
  AccelToAngles (not valid when upside down) VectorLength/1(roll (phi)) -> Mux7/1
  AccelToAngles (not valid when upside down) VectorLength/2(pitch (theta)) -> Mux7/2
  Switch3/1 -> Sum5/2
  (2^12)/3/1 -> Switch3/3
  Activate Calibration Accel Angles/1 -> Switch3/2
  Demux4/1 -> Trigonometric Function/1
  Demux4/2 -> Trigonometric Function/2
  Data Type Conversion/1 -> Demux4/1
  Trigonometric Function/1 -> MATLAB Function/2(b)
  MATLAB Function/1(anew) -> Terminator/1, Memory/1
  Memory/1 -> MATLAB Function/1(a)
  signconvention1/1 -> Height UltraSound/1, To Workspace3/1
  Sum1/1 -> Roll Pitch (Integrated Gyro + Accel Corrected)/1
  sign convention flip x axis/1 -> Data Type Conversion2/1
  Discrete-Time Integrator3/1 -> Memory3/1, Hold bias and scale after/1(ax ay az [raw]), AccelToAngles Vector length/1(ax ay az)
  Product5/1 -> Discrete-Time Integrator3/1
  Sum10/1 -> Product5/1
  1/tau/1 -> Product5/2
  Sum4/1 -> sign convention flip x axis/1
  "signconvention flip omega_{y,z}"/1 -> Data Type Conversion1/1
  Memory3/1 -> Sum10/2
  Data Type Conversion2/1 -> Sum10/1
  Mux1/1 -> Moving Average Filter/1(In)
  Discrete-Time Integrator1/1 -> Memory4/1, Sum/1, Moving Average Filter1/1(In)
  Product2/1 -> Discrete-Time Integrator1/1
  Sum3/1 -> Product2/1
  "1/tau "/1 -> Product2/2
  Memory4/1 -> Sum3/2
  Data Type Conversion1/1 -> Sum3/1
  Mux7/1 -> Sum5/1
  Memory6/1 -> Omega To d/dt Lambda/2(lambda_rpy), Sum8/1
  Sum5/1 -> Sum8/2, To Workspace10/1, RP Accel/1, Sum2/2
  SensorToRadials1/1 -> Sum7/2
  Sum7/1 -> Discrete-Time Integrator/1
  Sum8/1 -> SensorToRadials1/1  "(lambda - lambda_accel)"
  Discrete-Time Integrator/1 -> To Workspace7/1, Sum1/1, Sum2/1, Memory6/1
  Moving Average Filter/1(Out) -> Hold bias and scale after/2(roll pitch norm)
  Manual Switch/1 -> Sum1/2
  gain2/1 -> Manual Switch/2
  Hold Calibration Signal/1 -> Manual Switch2/1
  Manual Switch2/1 -> Hold the bias/2(hold signal), Discrete-Time Integrator/2, Hold bias and scale after/3(hold signal)
  gain3/1 -> Manual Switch1/1
  gain4/1 -> Manual Switch1/2
  Manual Switch1/1 -> Manual Switch2/2

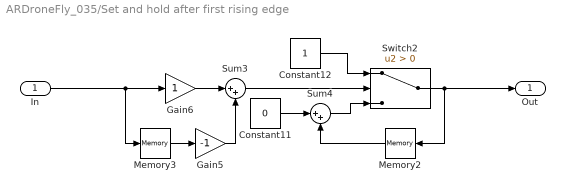
== system ARDroneFly_035/Set and hold after first rising edge ==
  In : Inport
  Constant11 : Constant  Value=0
  Constant12 : Constant
  Gain5 : Gain  Gain=-1
  Gain6 : Gain
  Memory2 : Memory
  Memory3 : Memory  X0=1
  Sum3 : Sum  Inputs=|++
  Sum4 : Sum  Inputs=|++
  Switch2 : Switch  Criteria=u2 > Threshold
  Out : Outport
  wires:
  Sum3/1 -> Switch2/2
  Constant12/1 -> Switch2/1
  Constant11/1 -> Sum4/1
  Memory2/1 -> Sum4/2
  Sum4/1 -> Switch2/3
  Switch2/1 -> Out/1, Memory2/1
  Gain6/1 -> Sum3/1
  Memory3/1 -> Gain5/1
  Gain5/1 -> Sum3/2
  In/1 -> Gain6/1, Memory3/1

== system ARDroneFly_035/Setpoint To Pilot Frame ==
  Setpoint : Inport
  yaw : Inport  Port=2
  Demux : Demux  Outputs=6
  Mux4 : Mux  Inputs=6
  To Pilot Frame : MATLAB Function  TreatAsAtomicUnit=on
  To Pilot Frame1 : MATLAB Function  TreatAsAtomicUnit=on
  Setpoint pilot frame : Outport
  wires:
  Demux/1 -> To Pilot Frame/1(Xa)  "x"
  Demux/2 -> To Pilot Frame/2(Ya)  "y"
  Demux/3 -> Mux4/3  "z"
  Setpoint/1 -> Demux/1
  To Pilot Frame/1(Xb) -> Mux4/1
  Mux4/1 -> Setpoint pilot frame/1
  To Pilot Frame/2(Yb) -> Mux4/2
  To Pilot Frame1/1(Xb) -> Mux4/5
  To Pilot Frame1/2(Yb) -> Mux4/6
  Demux/5 -> To Pilot Frame1/1(Xa)  "u"
  Demux/6 -> To Pilot Frame1/2(Ya)  "v"
  Demux/4 -> Mux4/4  "yaw"
  yaw/1 -> To Pilot Frame/3(yaw), To Pilot Frame1/3(yaw)

== system ARDroneFly_035/States To Pilot Frame ==
  State : Inport
  Demux : Demux  Outputs=12
  Mux4 : Mux  Inputs=12
  To Pilot Frame : MATLAB Function  TreatAsAtomicUnit=on
  To Pilot Frame1 : MATLAB Function  TreatAsAtomicUnit=on
  State pilot frame : Outport
  wires:
  To Pilot Frame/2(Yb) -> Mux4/2
  Mux4/1 -> State pilot frame/1
  To Pilot Frame/1(Xb) -> Mux4/1
  To Pilot Frame1/1(Xb) -> Mux4/7
  To Pilot Frame1/2(Yb) -> Mux4/8
  State/1 -> Demux/1
  Demux/12 -> Mux4/12  "omega_z"
  Demux/11 -> Mux4/11  "omega_y"
  Demux/10 -> Mux4/10  "omega_x"
  Demux/9 -> Mux4/9  "w"
  Demux/8 -> To Pilot Frame1/2(Ya)  "v"
  Demux/5 -> Mux4/5  "pitch"
  Demux/4 -> Mux4/4  "roll"
  Demux/3 -> Mux4/3  "z"
  Demux/2 -> To Pilot Frame/2(Ya)  "y"
  Demux/1 -> To Pilot Frame/1(Xa)  "x"
  Demux/6 -> To Pilot Frame1/3(yaw), To Pilot Frame/3(yaw), Mux4/6  "yaw"
  Demux/7 -> To Pilot Frame1/1(Xa)  "u"

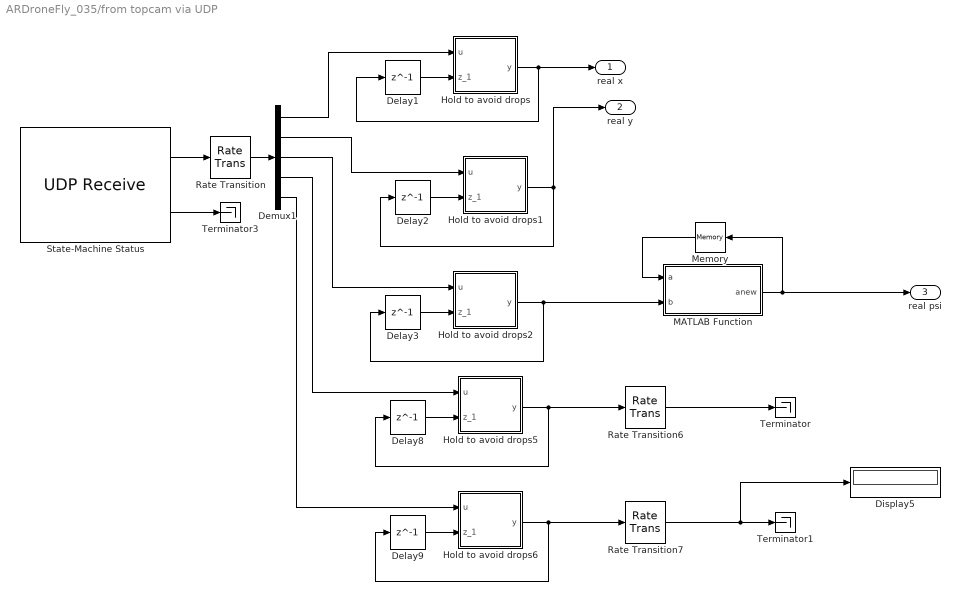
== system ARDroneFly_035/from topcam via UDP ==
  Delay{1..3,8..9} (5 alike) : Delay  DelayLength=1  InitialCondition=0
  Demux1 : Demux  Outputs=5
  Display5 : Display
  Hold to avoid drops : MATLAB Function  TreatAsAtomicUnit=on
  Hold to avoid drops1 : MATLAB Function  TreatAsAtomicUnit=on
  Hold to avoid drops2 : MATLAB Function  TreatAsAtomicUnit=on
  Hold to avoid drops5 : MATLAB Function  TreatAsAtomicUnit=on
  Hold to avoid drops6 : MATLAB Function  TreatAsAtomicUnit=on
  MATLAB Function : MATLAB Function  TreatAsAtomicUnit=on
  Memory : Memory
  Rate Transition : RateTransition
  Rate Transition6 : RateTransition
  Rate Transition7 : RateTransition
  State-Machine Status : dspnetwork/UDP Receive  localURL='0.0.0.0'  localPort=24000  remoteURL='192.168.1.1'  remotePort=-1  recvBufferSize=8192  dims=5  signalDatatype=double  isVarSize=off  showBlockingTime=on  blockingTime=0  sampletime=-1  blockPlatform=LINUX
  Terminator : Terminator
  Terminator1 : Terminator
  Terminator3 : Terminator
  real x : Outport
  "real y " : Outport  Port=2
  real psi : Outport  Port=3
  wires:
  Delay1/1 -> Hold to avoid drops/2(z_1)
  Demux1/1 -> Hold to avoid drops/1(u)
  Delay2/1 -> Hold to avoid drops1/2(z_1)
  Hold to avoid drops1/1(y) -> "real y "/1, Delay2/1
  Demux1/2 -> Hold to avoid drops1/1(u)
  State-Machine Status/2 -> Terminator3/1
  State-Machine Status/1 -> Rate Transition/1
  Rate Transition/1 -> Demux1/1
  Hold to avoid drops/1(y) -> Delay1/1, real x/1
  Delay8/1 -> Hold to avoid drops5/2(z_1)
  Hold to avoid drops5/1(y) -> Rate Transition6/1, Delay8/1
  Demux1/4 -> Hold to avoid drops5/1(u)
  Rate Transition6/1 -> Terminator/1
  Delay9/1 -> Hold to avoid drops6/2(z_1)
  Hold to avoid drops6/1(y) -> Rate Transition7/1, Delay9/1
  Demux1/5 -> Hold to avoid drops6/1(u)
  Rate Transition7/1 -> Terminator1/1, Display5/1
  Delay3/1 -> Hold to avoid drops2/2(z_1)
  Demux1/3 -> Hold to avoid drops2/1(u)
  Hold to avoid drops2/1(y) -> Delay3/1, MATLAB Function/2(b)
  Memory/1 -> MATLAB Function/1(a)
  MATLAB Function/1(anew) -> Memory/1, real psi/1

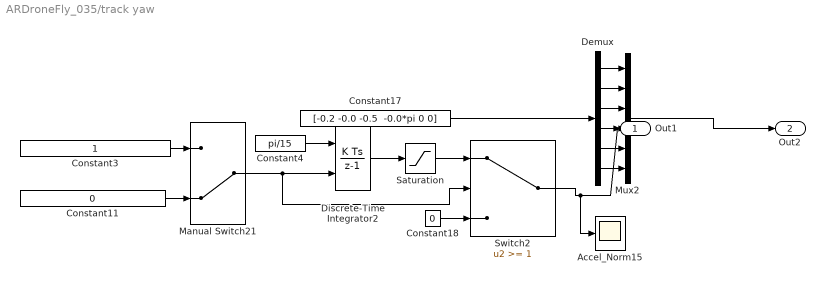
== system ARDroneFly_035/track yaw ==
  Accel_Norm15 : Scope
      settings: YMin=0  YMax=3.5  SaveName=Accel_P13
  Constant11 : Constant  Value=0
  Constant17 : Constant  Value="[-0.2 -0.0 -0.5  -0.0*pi 0 0]"
  Constant18 : Constant  Value=0
  Constant3 : Constant
  Constant4 : Constant  Value=pi/15
  Demux : Demux  Outputs=6
  Discrete-Time Integrator2 : DiscreteIntegrator  ExternalReset=rising  InitialConditionSetting=State (most efficient)  SampleTime=-1
  Manual Switch21 : ManualSwitch  CurrentSetting=0
  Mux2 : Mux  Inputs=6
  Saturation : Saturate  UpperLimit=pi*0.5  LowerLimit=0
  Switch2 : Switch  Threshold=1
  Out1 : Outport
  Out2 : Outport  Port=2
  wires:
  Constant3/1 -> Manual Switch21/1
  Constant11/1 -> Manual Switch21/2
  Demux/1 -> Mux2/1
  Demux/2 -> Mux2/2
  Demux/3 -> Mux2/3
  Demux/5 -> Mux2/5
  Demux/6 -> Mux2/6
  Mux2/1 -> Out2/1
  Constant4/1 -> Discrete-Time Integrator2/1
  Discrete-Time Integrator2/1 -> Saturation/1
  Constant17/1 -> Demux/1
  Manual Switch21/1 -> Switch2/2, Discrete-Time Integrator2/2
  Switch2/1 -> Accel_Norm15/1, Mux2/4
  Saturation/1 -> Switch2/1
  Constant18/1 -> Switch2/3
  Demux/4 -> Out1/1

== system ARDroneFly_035/Battery Check/Hold forever after rising edge ==
  in : Inport
  reset : Inport  Port=2
  Constant1 : Constant
  Constant2 : Constant  Value=0
  Constant3 : Constant  Value=0
  Memory : Memory
  Sum : Sum  Inputs=|++
  Switch1 : Switch  Threshold=1
  Switch3 : Switch  Threshold=1
  out : Outport
  wires:
  Switch3/1 -> Switch1/2
  Sum/1 -> Switch3/3
  in/1 -> Sum/1
  Switch1/1 -> out/1, Memory/1
  Constant3/1 -> Switch3/1
  reset/1 -> Switch3/2
  Constant2/1 -> Switch1/3
  Constant1/1 -> Switch1/1
  Memory/1 -> Sum/2

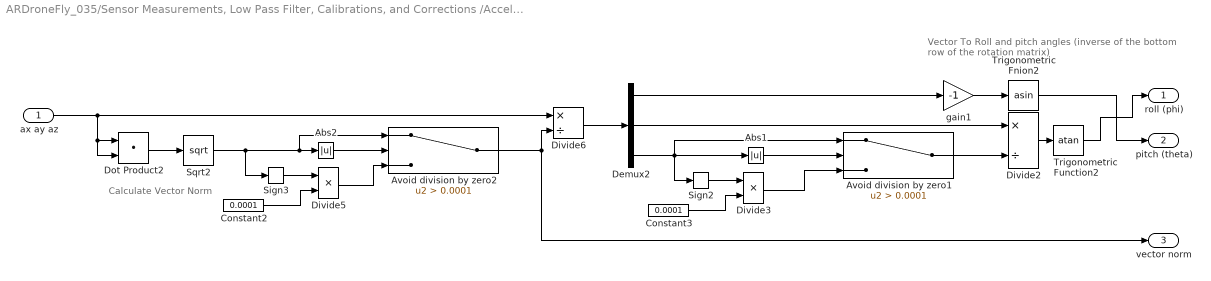
== system ARDroneFly_035/Sensor Measurements, Low Pass Filter, Calibrations, and Corrections /AccelToAngles Vector length ==
  note: Vector To Roll and pitch angles
      | (inverse of the bottom row of the rotation matrix)
  note: Calculate Vector Norm
  ax ay az : Inport
  Abs1 : Abs
  Abs2 : Abs
  Avoid division by zero1 : Switch  Criteria=u2 > Threshold  Threshold=0.0001
  Avoid division by zero2 : Switch  Criteria=u2 > Threshold  Threshold=0.0001
  Constant2 : Constant  Value=0.0001
  Constant3 : Constant  Value=0.0001
  Demux2 : Demux  Outputs=3
  Divide2 : Product  Inputs=*/
  Divide3 : Product  Inputs=**
  Divide5 : Product  Inputs=**
  Divide6 : Product  Inputs=*/
  Dot Product2 : DotProduct  InputSameDT=on  OutDataTypeStr=Inherit: Inherit via internal rule
  Sign2 : Signum
  Sign3 : Signum
  Sqrt2 : Sqrt  SaturateOnIntegerOverflow=on
  Trigonometric Fnion2 : Trigonometry  Operator=asin
  Trigonometric Function2 : Trigonometry  Operator=atan
  gain1 : Gain  Gain=-1
  roll (phi) : Outport
  pitch (theta) : Outport  Port=2
  vector norm : Outport  Port=3
  wires:
  Divide2/1 -> Trigonometric Function2/1
  Demux2/2 -> Divide2/1
  Demux2/1 -> gain1/1
  Divide6/1 -> Demux2/1
  gain1/1 -> Trigonometric Fnion2/1
  Dot Product2/1 -> Sqrt2/1
  ax ay az/1 -> Dot Product2/1, Dot Product2/2, Divide6/1
  Avoid division by zero1/1 -> Divide2/2
  Abs1/1 -> Avoid division by zero1/2
  Demux2/3 -> Sign2/1, Avoid division by zero1/1, Abs1/1
  Divide3/1 -> Avoid division by zero1/3
  Constant3/1 -> Divide3/2
  Sign2/1 -> Divide3/1
  Avoid division by zero2/1 -> vector norm/1, Divide6/2
  Abs2/1 -> Avoid division by zero2/2
  Sqrt2/1 -> Sign3/1, Abs2/1, Avoid division by zero2/1
  Constant2/1 -> Divide5/2
  Sign3/1 -> Divide5/1
  Divide5/1 -> Avoid division by zero2/3
  Trigonometric Fnion2/1 -> pitch (theta)/1
  Trigonometric Function2/1 -> roll (phi)/1

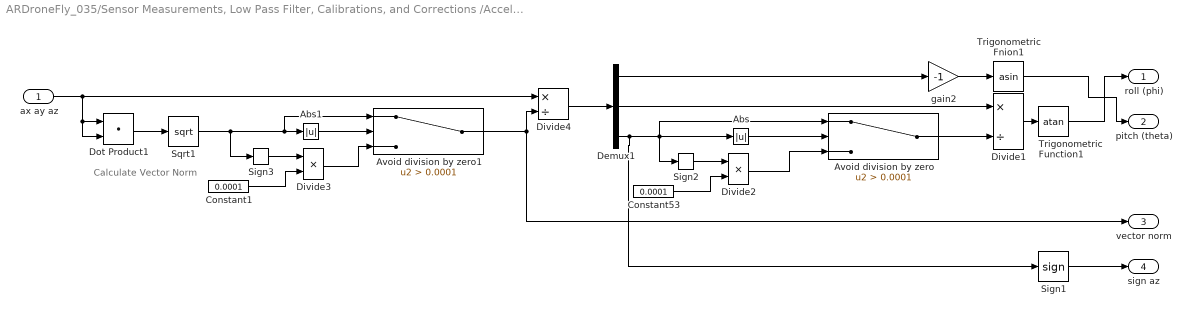
== system ARDroneFly_035/Sensor Measurements, Low Pass Filter, Calibrations, and Corrections /AccelToAngles (not valid when upside down) VectorLength ==
  note: Calculate Vector Norm
  ax ay az : Inport
  Abs : Abs
  Abs1 : Abs
  Avoid division by zero : Switch  Criteria=u2 > Threshold  Threshold=0.0001
  Avoid division by zero1 : Switch  Criteria=u2 > Threshold  Threshold=0.0001
  Constant1 : Constant  Value=0.0001
  Constant53 : Constant  Value=0.0001
  Demux1 : Demux  Outputs=3
  Divide1 : Product  Inputs=*/
  Divide2 : Product  Inputs=**
  Divide3 : Product  Inputs=**
  Divide4 : Product  Inputs=*/
  Dot Product1 : DotProduct  InputSameDT=on  OutDataTypeStr=Inherit: Inherit via internal rule
  Sign1 : Signum
  Sign2 : Signum
  Sign3 : Signum
  Sqrt1 : Sqrt  SaturateOnIntegerOverflow=on
  Trigonometric Fnion1 : Trigonometry  Operator=asin
  Trigonometric Function1 : Trigonometry  Operator=atan
  gain2 : Gain  Gain=-1
  roll (phi) : Outport
  pitch (theta) : Outport  Port=2
  vector norm : Outport  Port=3
  sign az : Outport  Port=4
  wires:
  Trigonometric Fnion1/1 -> pitch (theta)/1
  Trigonometric Function1/1 -> roll (phi)/1
  Divide1/1 -> Trigonometric Function1/1
  Demux1/2 -> Divide1/1
  Demux1/1 -> gain2/1
  Divide4/1 -> Demux1/1
  gain2/1 -> Trigonometric Fnion1/1
  Dot Product1/1 -> Sqrt1/1
  ax ay az/1 -> Dot Product1/1, Dot Product1/2, Divide4/1
  Sign1/1 -> sign az/1
  Avoid division by zero/1 -> Divide1/2
  Abs/1 -> Avoid division by zero/2
  Demux1/3 -> Sign1/1, Sign2/1, Avoid division by zero/1, Abs/1
  Divide2/1 -> Avoid division by zero/3
  Constant53/1 -> Divide2/2
  Sign2/1 -> Divide2/1
  Avoid division by zero1/1 -> Divide4/2, vector norm/1
  Abs1/1 -> Avoid division by zero1/2
  Sqrt1/1 -> Sign3/1, Abs1/1, Avoid division by zero1/1
  Constant1/1 -> Divide3/2
  Sign3/1 -> Divide3/1
  Divide3/1 -> Avoid division by zero1/3

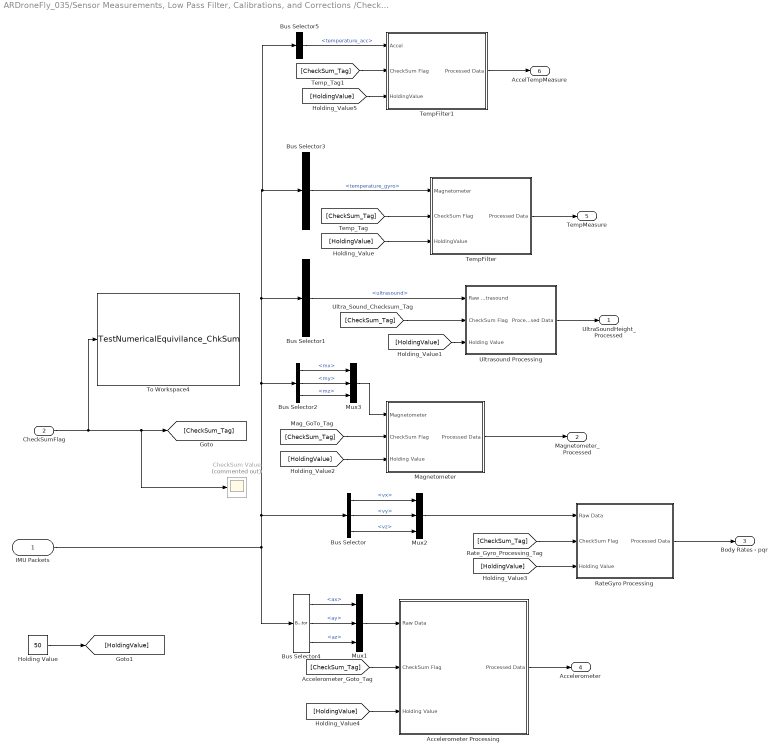
== system ARDroneFly_035/Sensor Measurements, Low Pass Filter, Calibrations, and Corrections /CheckSum Pre-Processing ==
  IMU Packets : Inport
  CheckSumFlag : Inport  Port=2
  Accelerometer Processing : Subsystem
  Bus Selector : BusSelector  OutputSignals=vx,vy,vz
  Bus Selector1 : BusSelector  OutputSignals=ultrasound
  Bus Selector2 : BusSelector  OutputSignals=mx,my,mz
  Bus Selector3 : BusSelector  OutputSignals=temperature_gyro
  Bus Selector4 : BusSelector  OutputSignals=ax,ay,az
  Bus Selector5 : BusSelector  OutputSignals=temperature_acc
  CheckSum Value : Scope  Commented=on
      settings: YMin=0  YMax=2500  SaveName=CheckSum
  Holding Value : Constant  Value=50
  Magnetometer : Subsystem
  Mux1 : Mux  Inputs=3
  Mux2 : Mux  Inputs=3
  Mux3 : Mux  Inputs=3
  RateGyro Processing : Subsystem
  TempFilter : Subsystem
  TempFilter1 : Subsystem
  To Workspace4 : ToWorkspace  VariableName=TestNumericalEquivilance_ChkSum  SaveFormat=Structure With Time  SampleTime=-1
  Ultrasound Processing : Subsystem
  UltraSoundHeight_Processed : Outport
  Magnetometer_Processed : Outport  Port=2
  Body Rates - pqr : Outport  Port=3
  Accelerometer : Outport  Port=4
  TempMeasure : Outport  Port=5
  AccelTempMeasure : Outport  Port=6
  wires:
  Bus Selector5/1 -> TempFilter1/1(Accel)  "<temperature_acc>"
  [HoldingValue] -> TempFilter1/3(HoldingValue)
  [CheckSum_Tag] -> TempFilter1/2(CheckSum Flag)
  TempFilter1/1(Processed Data) -> AccelTempMeasure/1
  Mux3/1 -> Magnetometer/1(Magnetometer)
  Holding Value/1 -> [HoldingValue]
  [HoldingValue] -> Accelerometer Processing/3(Holding Value)
  [HoldingValue] -> RateGyro Processing/3(Holding Value)
  [HoldingValue] -> Magnetometer/3(Holding Value)
  [HoldingValue] -> Ultrasound Processing/3(Holding Value)
  [HoldingValue] -> TempFilter/3(HoldingValue)
  [CheckSum_Tag] -> TempFilter/2(CheckSum Flag)
  TempFilter/1(Processed Data) -> TempMeasure/1
  Bus Selector3/1 -> TempFilter/1(Magnetometer)  "<temperature_gyro>"
  Bus Selector/3 -> Mux2/3  "<vz>"
  Bus Selector/2 -> Mux2/2  "<vy>"
  Bus Selector/1 -> Mux2/1  "<vx>"
  Ultrasound Processing/1(Processed Data) -> UltraSoundHeight_Processed/1
  [CheckSum_Tag] -> Accelerometer Processing/2(CheckSum Flag)
  Magnetometer/1(Processed Data) -> Magnetometer_Processed/1
  [CheckSum_Tag] -> Magnetometer/2(CheckSum Flag)
  Bus Selector2/3 -> Mux3/3  "<mz>"
  Bus Selector2/2 -> Mux3/2  "<my>"
  Bus Selector2/1 -> Mux3/1  "<mx>"
  RateGyro Processing/1(Processed Data) -> Body Rates - pqr/1
  [CheckSum_Tag] -> RateGyro Processing/2(CheckSum Flag)
  Mux2/1 -> RateGyro Processing/1(Raw Data)
  Accelerometer Processing/1(Processed Data) -> Accelerometer/1
  [CheckSum_Tag] -> Ultrasound Processing/2(CheckSum Flag)
  Mux1/1 -> Accelerometer Processing/1(Raw Data)
  Bus Selector4/3 -> Mux1/3  "<az>"
  Bus Selector4/2 -> Mux1/2  "<ay>"
  Bus Selector4/1 -> Mux1/1  "<ax>"
  IMU Packets/1 -> Bus Selector4/1, Bus Selector2/1, Bus Selector1/1, Bus Selector3/1, Bus Selector5/1, Bus Selector/1
  CheckSumFlag/1 -> CheckSum Value/1, [CheckSum_Tag], To Workspace4/1
  Bus Selector1/1 -> Ultrasound Processing/1(Raw Ultrasound)  "<ultrasound>"

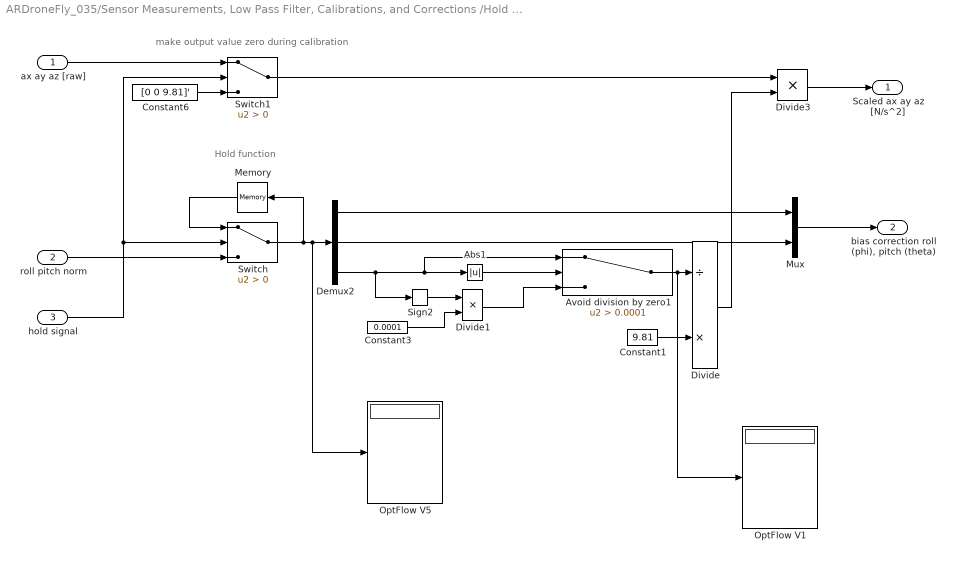
== system ARDroneFly_035/Sensor Measurements, Low Pass Filter, Calibrations, and Corrections /Hold bias and scale after ==
  note: Hold function
  note: make output value zero during calibration
  ax ay az [raw] : Inport
  roll pitch norm : Inport  Port=2
  hold signal : Inport  Port=3
  Abs1 : Abs
  Avoid division by zero1 : Switch  Criteria=u2 > Threshold  Threshold=0.0001
  Constant1 : Constant  Value=9.81
  Constant3 : Constant  Value=0.0001
  Constant6 : Constant  Value=[0 0 9.81]'
  Demux2 : Demux  Outputs=3
  Divide : Product  Inputs=/*
  Divide1 : Product  Inputs=**
  Divide3 : Product  Inputs=**
  Memory : Memory  X0=[0 0 9.81]
  Mux : Mux  Inputs=2
  OptFlow V1 : Display
  OptFlow V5 : Display
  Sign2 : Signum
  Switch : Switch  Criteria=u2 > Threshold
  Switch1 : Switch  Criteria=u2 > Threshold
  "Scaled ax ay az [N/s^2] " : Outport
  "bias correction roll (phi), pitch (theta)" : Outport  Port=2
  wires:
  ax ay az [raw]/1 -> Switch1/1
  Switch/1 -> OptFlow V5/1, Demux2/1, Memory/1
  Divide/1 -> Divide3/2
  hold signal/1 -> Switch/2, Switch1/2
  Divide3/1 -> "Scaled ax ay az [N/s^2] "/1
  Constant6/1 -> Switch1/3
  Constant1/1 -> Divide/2
  Memory/1 -> Switch/1
  roll pitch norm/1 -> Switch/3
  Demux2/2 -> Mux/2
  Demux2/1 -> Mux/1
  Mux/1 -> "bias correction roll (phi), pitch (theta)"/1
  Switch1/1 -> Divide3/1
  Abs1/1 -> Avoid division by zero1/2
  Demux2/3 -> Avoid division by zero1/1, Abs1/1, Sign2/1
  Divide1/1 -> Avoid division by zero1/3
  Constant3/1 -> Divide1/2
  Sign2/1 -> Divide1/1
  Avoid division by zero1/1 -> OptFlow V1/1, Divide/1

== system ARDroneFly_035/Sensor Measurements, Low Pass Filter, Calibrations, and Corrections /Hold the bias ==
  bias wx wy wz : Inport
  hold signal : Inport  Port=2
  Memory : Memory
  Switch : Switch  Criteria=u2 > Threshold
  " holded bias wx wy wz" : Outport
  wires:
  bias wx wy wz/1 -> Switch/3
  Memory/1 -> Switch/1
  Switch/1 -> Memory/1, " holded bias wx wy wz"/1
  hold signal/1 -> Switch/2

== system ARDroneFly_035/Sensor Measurements, Low Pass Filter, Calibrations, and Corrections /Moving Average Filter ==
  In : Inport
  ratio new/old value : Inport  Port=2
  " " : Constant
  Memory1 : Memory  X0=[0 0 9.81]
  Product1 : Product  Inputs=**
  Product2 : Product  Inputs=**
  Sum3 : Sum  Inputs=|++
  Sum5 : Sum  Inputs=-+|
  Out : Outport
  wires:
  Memory1/1 -> Product2/2
  Product1/1 -> Sum3/1
  Sum3/1 -> Memory1/1, Out/1
  Sum5/1 -> Product2/1
  In/1 -> Product1/1
  " "/1 -> Sum5/2
  ratio new/old value/1 -> Sum5/1, Product1/2
  Product2/1 -> Sum3/2

== system ARDroneFly_035/Sensor Measurements, Low Pass Filter, Calibrations, and Corrections /Moving Average Filter1 ==
  In : Inport
  ratio new/old value : Inport  Port=2
  " " : Constant
  Memory1 : Memory
  Product1 : Product  Inputs=**
  Product2 : Product  Inputs=**
  Sum3 : Sum  Inputs=|++
  Sum5 : Sum  Inputs=-+|
  Out : Outport
  wires:
  ratio new/old value/1 -> Product1/2, Sum5/1
  " "/1 -> Sum5/2
  In/1 -> Product1/1
  Sum5/1 -> Product2/1
  Sum3/1 -> Memory1/1, Out/1
  Product1/1 -> Sum3/1
  Memory1/1 -> Product2/2
  Product2/1 -> Sum3/2
